simulink subsystem "LocalizationSystem"  (R2024b)
settings: Solver=VariableStepAuto  StartTime=0.0  StopTime=10.0  RelTol=1e-3
undefined symbols (not defined in the file or in its folder): DiscIntNeverNeededParam
libraries: robotcorelib x3, simulink x1
settings Model: Creator=Sasha  LastModifiedBy=vince

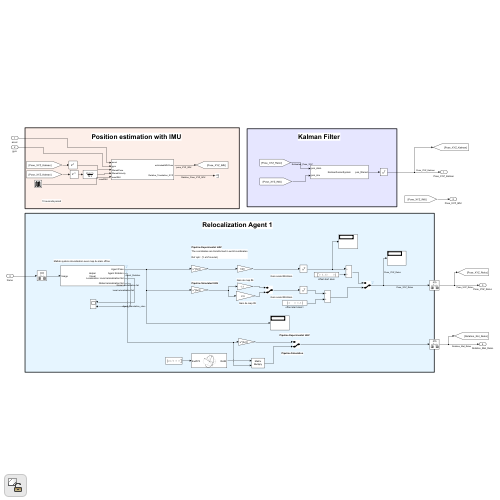
[thumbnail: Simulink's stored preview of the top-level diagram]
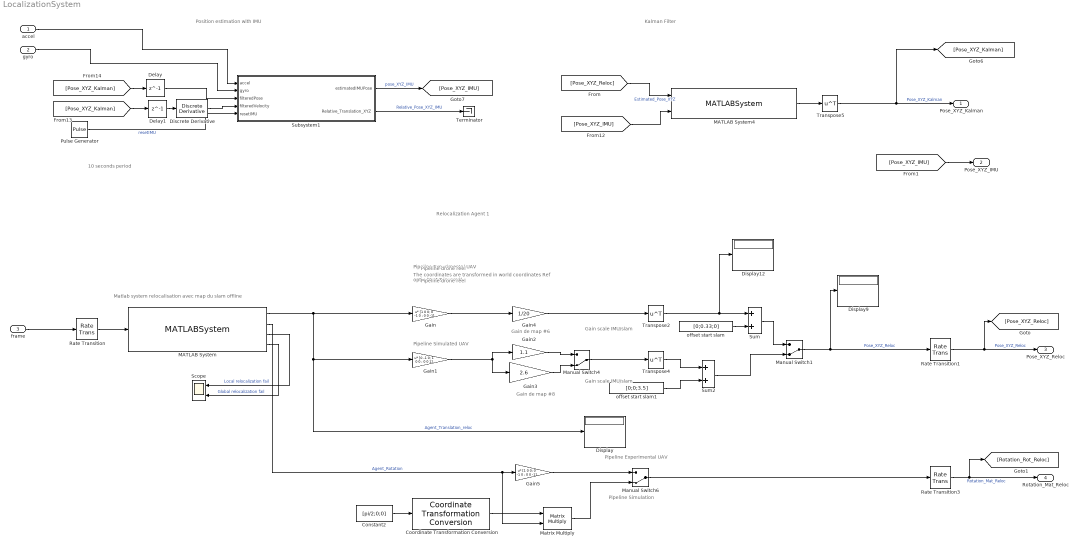
== system LocalizationSystem ==
  note: Gain de map #6
  note: Pipeline Experimental UAV
  note: Matlab system relocalisation avec map du slam offline
  note: Gain scale IMU/slam
  note: The coordinates are transformed in world coordinates
      |
      | Ref opti : (Y et Z inversé)
  note: Gain scale IMU/slam
  note: Pipeline drone réel
  note: Pipeline drone réel
  note: Pipeline Simulated UAV
  note: Gain de map #8
  note: 10 seconds period
  note: Relocalization Agent 1
  note: Position estimation with IMU
  note: Kalman Filter
  note: Pipeline Experimental UAV
  note: Pipeline Simulation
  accel : Inport
  gyro : Inport  Port=2
  frame : Inport  Port=3
  Constant2 : Constant  Value=[pi/2;0;0]
  Coordinate Transformation Conversion : robotcorelib/Coordinate Transformation Conversion  InputRepresentation=Euler Angles  InputEulerSequence=ZYX  ShowTrVecInputPort=on  OutputRepresentation=Rotation Matrix  OutputEulerSequence=ZYX  ShowTrVecOutputPort=on  SimulateUsing=Code generation
  Delay : Delay  DelayLength=1  InitialCondition=[0;0;0]
  Delay1 : Delay  DelayLength=1  InitialCondition=[0;0;0]
  Discrete Derivative : simulink/Discrete/Discrete Derivative  gainval=1.0  ICPrevScaledInput=0.0  OutMin=[]  OutMax=[]  OutDataType=fixdt(1, 16)  OutScaling=2^-10  DoSatur=off
  Display : Display
  Display12 : Display
  Display9 : Display
  Gain : Gain  Gain=[1 0 0; 0 -1 0 ; 0 0 -1]  Multiplication=Matrix(u*K)
  Gain1 : Gain  Gain=[0 -1 0; 1 0 0 ; 0 0 1]  Multiplication=Matrix(u*K)
  Gain2 : Gain  Gain=1.1
  Gain3 : Gain  Gain=2.6
  Gain4 : Gain  Gain=1/20
  Gain5 : Gain  Gain=[1 0 0; 0 -1 0 ; 0 0 -1]  Multiplication=Matrix(u*K)
  MATLAB System : MATLABSystem  System=Modif_of_HelperVisualLocalizationSystem  FocalLength=[1109,1109]  PrincipalPoint=[640,360]  ImageSize=[720,1280]  ScaleFactor=1.2  NumLevels=8  NumPoints=2000  XLim=[-100 100]  YLim=[-100 100]  ZLim=[-100 100]  SampleTime=0.1  ScenariosDirectory=C:\Users\vince\Documents\SEN5\CollaborativeSLAM\Scenarios  ScenarioName=8
      mask Type: Modif_of_HelperVisualLocalizationSystem
      mask Display:
      | disp(['Helper' char(10) 'Visual' char(10) 'Localization']);
      | port_label('input',1,'Image');
      | port_label('output',1,'Agent Pose');
      | port_label('output',2,'Agent Rotation');
      | port_label('output',3,'Local relocalization fail');
      | port_label('output',4,'Global relocalization fail');
  MATLAB System4 : MATLABSystem  System=KalmanFusionSystem  dt=0.1  noise_std=0.1  Q=0.001 * eye( 6 )  R=diag( [ 0.3, 0.3, 0.3, 0.1, 0.1, 0.1 ] )  SimulateUsing=Interpreted execution
      mask Type: KalmanFusionSystem
      mask Display:
      | disp('KalmanFusionSystem');
      | port_label('input',1,'pos_slam');
      | port_label('input',2,'pos_imu');
      | port_label('output',1,'pos_filtered');
  Manual Switch1 : ManualSwitch  CurrentSetting=0
  Manual Switch4 : ManualSwitch  CurrentSetting=0
  Manual Switch6 : ManualSwitch  CurrentSetting=0
  Matrix Multiply : Product  Multiplication=Matrix(*)
  Pulse Generator : DiscretePulseGenerator  PulseType=Time based  Period=0.05  PulseWidth=50
  Rate Transition : RateTransition
  Rate Transition1 : RateTransition
  Rate Transition3 : RateTransition
  Scope : Scope  NumInputPorts=2
  Subsystem1 : Subsystem
  Sum : Sum
  Sum2 : Sum
  Terminator : Terminator
  Transpose2 : Math  Operator=transpose
  Transpose4 : Math  Operator=transpose
  Transpose5 : Math  Operator=transpose
  offset start slam : Constant  Value=[0;0.33;0]
  offset start slam1 : Constant  Value=[0;0;3.5]
  Pose_XYZ_Kalman : Outport
  Pose_XYZ_IMU : Outport  Port=2
  Pose_XYZ_Reloc : Outport  Port=3
  Rotation_Mat_Reloc : Outport  Port=4
  wires:
  Rate Transition1/1 -> Pose_XYZ_Reloc/1, [Pose_XYZ_Reloc]  "Pose_XYZ_Reloc"
  frame/1 -> Rate Transition/1
  [Pose_XYZ_Kalman] -> Delay/1
  Transpose2/1 -> Sum/1, Display12/1
  Sum2/1 -> Manual Switch1/2
  Delay/1 -> Subsystem1/3(filteredPose)
  Gain/1 -> Gain4/1
  Gain5/1 -> Manual Switch6/1
  Gain2/1 -> Manual Switch4/1
  Coordinate Transformation Conversion/1 -> Matrix Multiply/1
  offset start slam1/1 -> Sum2/2
  MATLAB System/2 -> Gain5/1, Matrix Multiply/2  "Agent_Rotation"
  gyro/1 -> Subsystem1/2(gyro)
  Constant2/1 -> Coordinate Transformation Conversion/1
  MATLAB System/1 -> Gain/1, Display/1, Gain1/1  "Agent_Translation_reloc"
  Transpose4/1 -> Sum2/1
  Manual Switch6/1 -> Rate Transition3/1
  Subsystem1/1(estimatedIMUPose) -> [Pose_XYZ_IMU]  "pose_XYZ_IMU"
  MATLAB System4/1 -> Transpose5/1
  Gain4/1 -> Transpose2/1
  Subsystem1/2(Relative_Translation_XYZ) -> Terminator/1  "Relative_Pose_XYZ_IMU"
  [Pose_XYZ_Kalman] -> Delay1/1
  Manual Switch1/1 -> Rate Transition1/1, Display9/1  "Pose_XYZ_Reloc"
  MATLAB System/4 -> Scope/2  "Global relocalization fail"
  accel/1 -> Subsystem1/1(accel)
  Rate Transition/1 -> MATLAB System/1
  offset start slam/1 -> Sum/2
  Rate Transition3/1 -> Rotation_Mat_Reloc/1, [Rotation_Rot_Reloc]  "Rotation_Mat_Reloc"
  Transpose5/1 -> [Pose_XYZ_Kalman], Pose_XYZ_Kalman/1  "Pose_XYZ_Kalman"
  Gain1/1 -> Gain2/1, Gain3/1
  Pulse Generator/1 -> Subsystem1/5(resetIMU)  "resetIMU"
  Matrix Multiply/1 -> Manual Switch6/2
  [Pose_XYZ_Reloc] -> MATLAB System4/1  "Estimated_Pose_XYZ"
  [Pose_XYZ_IMU] -> MATLAB System4/2
  Manual Switch4/1 -> Transpose4/1
  MATLAB System/3 -> Scope/1  "Local relocalization fail"
  Gain3/1 -> Manual Switch4/2
  Sum/1 -> Manual Switch1/1
  Delay1/1 -> Discrete Derivative/1
  Discrete Derivative/1 -> Subsystem1/4(filteredVelocity)
  [Pose_XYZ_IMU] -> Pose_XYZ_IMU/1

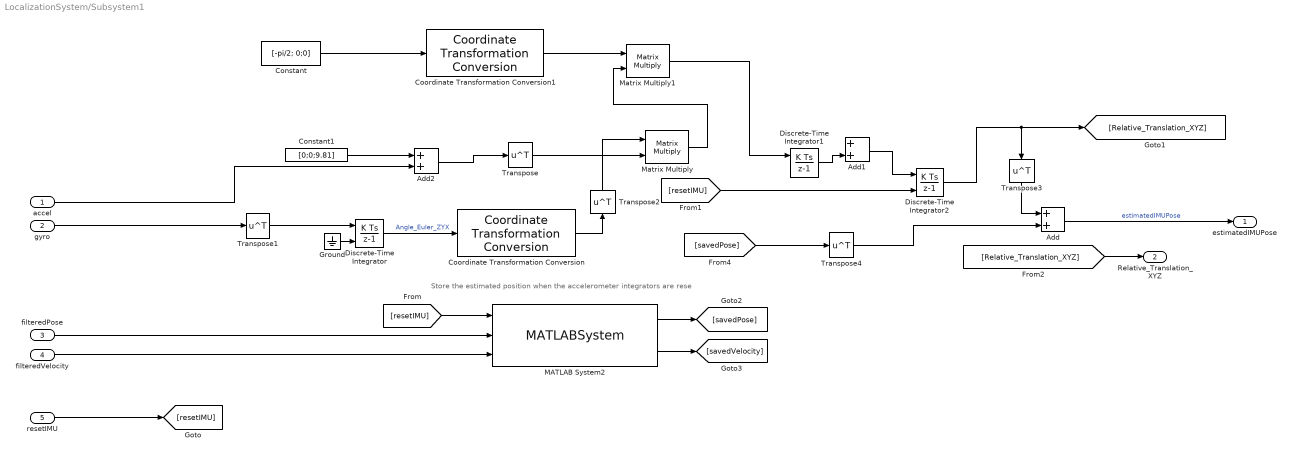
== system LocalizationSystem/Subsystem1 ==
  note: Store the estimated position when the accelerometer integrators are rese
  accel : Inport
  gyro : Inport  Port=2
  filteredPose : Inport  Port=3
  filteredVelocity : Inport  Port=4  PortDimensions=[3,1]
  resetIMU : Inport  Port=5
  Add : Sum
  Add1 : Sum
  Add2 : Sum
  Constant : Constant  Value=[-pi/2; 0;0]
  Constant1 : Constant  Value=[0;0;9.81]
  Coordinate Transformation Conversion : robotcorelib/Coordinate Transformation Conversion  InputRepresentation=Euler Angles  InputEulerSequence=ZYX  ShowTrVecInputPort=on  OutputRepresentation=Rotation Matrix  OutputEulerSequence=ZYX  ShowTrVecOutputPort=on  SimulateUsing=Code generation
  Coordinate Transformation Conversion1 : robotcorelib/Coordinate Transformation Conversion  InputRepresentation=Euler Angles  InputEulerSequence=ZYX  ShowTrVecInputPort=on  OutputRepresentation=Rotation Matrix  OutputEulerSequence=ZYX  ShowTrVecOutputPort=on  SimulateUsing=Code generation
  Discrete-Time Integrator : DiscreteIntegrator  ExternalReset=rising  SampleTime=-1  ICPrevOutput=DiscIntNeverNeededParam  ICPrevScaledInput=DiscIntNeverNeededParam
  Discrete-Time Integrator1 : DiscreteIntegrator  ExternalReset=rising  SampleTime=-1  ICPrevOutput=DiscIntNeverNeededParam  ICPrevScaledInput=DiscIntNeverNeededParam
  Discrete-Time Integrator2 : DiscreteIntegrator  ExternalReset=rising  SampleTime=-1  ICPrevOutput=DiscIntNeverNeededParam  ICPrevScaledInput=DiscIntNeverNeededParam
  Ground : Ground
  MATLAB System2 : MATLABSystem  System=IMUPoseMemory  SimulateUsing=Interpreted execution
      mask Type: IMUPoseMemory
      mask Display:
      | disp('IMUPoseMemory');
      | port_label('input',1,'resetImu');
      | port_label('input',2,'filteredPose');
      | port_label('input',3,'filteredVelocity');
      | port_label('output',1,'savedPose');
      | port_label('output',2,'savedVelocity');
  Matrix Multiply : Product  Multiplication=Matrix(*)
  Matrix Multiply1 : Product  Multiplication=Matrix(*)
  Transpose{,1..4} (5 alike) : Math  Operator=transpose
  estimatedIMUPose : Outport
  Relative_Translation_XYZ : Outport  Port=2
  wires:
  Matrix Multiply1/1 -> Discrete-Time Integrator1/1
  Matrix Multiply/1 -> Matrix Multiply1/2
  Transpose3/1 -> Add/1
  Add1/1 -> Discrete-Time Integrator2/1
  MATLAB System2/2 -> [savedVelocity]
  filteredVelocity/1 -> MATLAB System2/3
  [Relative_Translation_XYZ] -> Relative_Translation_XYZ/1
  Transpose2/1 -> Matrix Multiply/1
  Discrete-Time Integrator2/1 -> [Relative_Translation_XYZ], Transpose3/1
  Coordinate Transformation Conversion1/1 -> Matrix Multiply1/1
  Constant/1 -> Coordinate Transformation Conversion1/1
  gyro/1 -> Transpose1/1
  resetIMU/1 -> [resetIMU]
  accel/1 -> Add2/2
  MATLAB System2/1 -> [savedPose]
  [resetIMU] -> MATLAB System2/1
  Transpose4/1 -> Add/2
  Add2/1 -> Transpose/1
  Discrete-Time Integrator/1 -> Coordinate Transformation Conversion/1  "Angle_Euler_ZYX"
  Add/1 -> estimatedIMUPose/1  "estimatedIMUPose"
  Transpose/1 -> Matrix Multiply/2
  Coordinate Transformation Conversion/1 -> Transpose2/1
  [resetIMU] -> Discrete-Time Integrator2/2
  Ground/1 -> Discrete-Time Integrator/2
  Discrete-Time Integrator1/1 -> Add1/2
  Constant1/1 -> Add2/1
  [savedPose] -> Transpose4/1
  Transpose1/1 -> Discrete-Time Integrator/1
  filteredPose/1 -> MATLAB System2/2
